simulink model "state_space"  (R2023b)
settings: Solver=VariableStepAuto  StartTime=0.0  StopTime=8  RelTol=1e-3
undefined symbols (not defined in the file): A, B, C, D, d2, Kc, n2
settings Model: Creator=foderking  LastModifiedBy=foderking

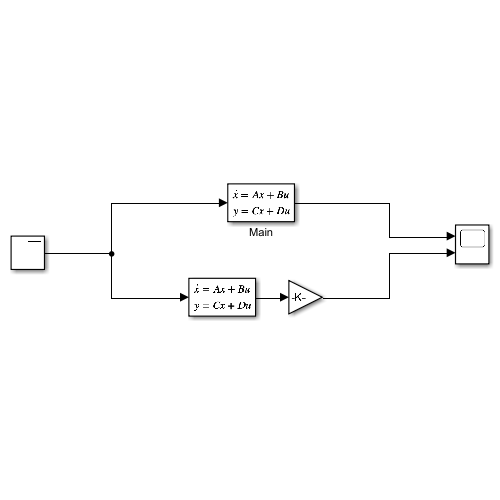
[thumbnail: Simulink's stored preview of the top-level diagram]
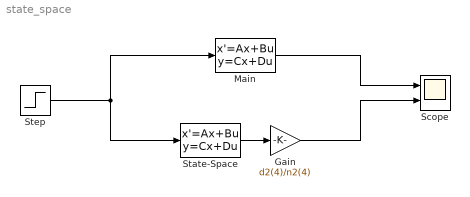
== system state_space ==
  Gain : Gain  Gain=d2(4)/n2(4)
  Main : StateSpace  A=A  B=B  C=C  D=D  InitialCondition=0
  Scope : Scope  NumInputPorts=2
  State-Space : StateSpace  A=A-B*Kc  B=B  C=C  D=D  InitialCondition=0
  Step : Step  Time=0  SampleTime=0
  wires:
  Step/1 -> Main/1, State-Space/1
  Main/1 -> Scope/1
  State-Space/1 -> Gain/1
  Gain/1 -> Scope/2
